simulink model "motor"  (R2021a)
settings: Solver=VariableStepAuto  StartTime=0.0  StopTime=0.05  FixedStep=0.01  RelTol=1e-3
InitFcn:
  | prop_init_set
settings Model: SimulationMode=accelerator  Creator=76568  LastModifiedBy=76568

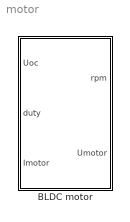
== system motor ==
  BLDC motor : Subsystem  mask{Kv=175, Rm=0.184}

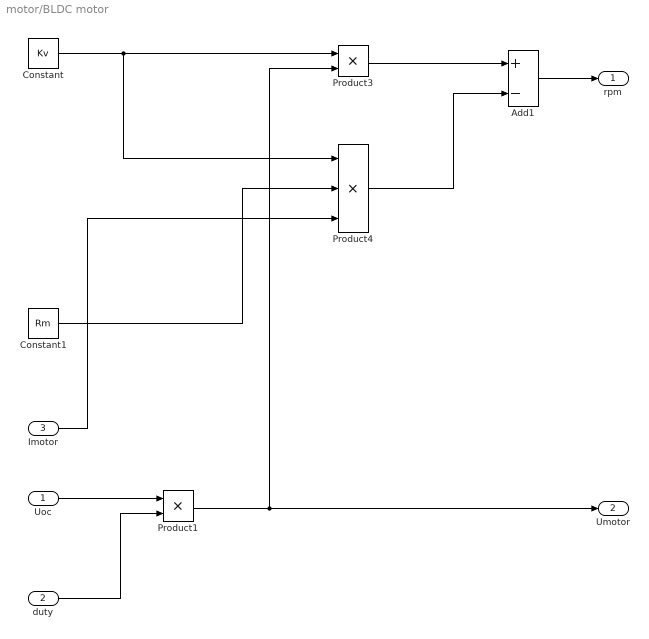
== system motor/BLDC motor ==
  Uoc : Inport
  duty : Inport  Port=2
  Imotor : Inport  Port=3
  Add1 : Sum  Inputs=+-
  Constant : Constant  Value=Kv
  Constant1 : Constant  Value=Rm
  Product1 : Product
  Product3 : Product  Inputs=**
  Product4 : Product  Inputs=***
  rpm : Outport
  Umotor : Outport  Port=2
  wires:
  Constant/1 -> Product4/1, Product3/1
  Product1/1 -> Product3/2, Umotor/1
  Constant1/1 -> Product4/2
  Product3/1 -> Add1/1
  Product4/1 -> Add1/2
  duty/1 -> Product1/2
  Add1/1 -> rpm/1
  Imotor/1 -> Product4/3
  Uoc/1 -> Product1/1
